simulink model "motor_model_9_az"  (R2018b)
settings: Solver=VariableStepAuto  StartTime=0.0  StopTime=1  RelTol=1e-7
model workspace (MAT data in the model file):
  A1 = 0.209333333333
  A2 = 0.0330526315789
  Ce = 0.27
  Cm = 0.36
  Jsumm = 7.5e-06
  K = 1000
  Kf = 0.1
  Km = 3.29
  Kn = 3.7
  L = 0.032
  Mn = 0.08
  R = 0.32
  T1 = 0.05
  T2 = 0.0001
  Te = 0.1
  Tm = 1.08
  Tpwm = 6.25e-05
  U = 27
  a = 0
  b = -2.09439510239
  c = 2.09439510239
  dt = 0.6
  dx = 3.14
  max = 3.14
  min = -3.14
  omega1 = 1.005
  omega2 = 6.28
  poles = 8
  target = 3.14
  w = 0.209333333333
libraries: simulink x2
settings Model: Creator=Sainquake  LastModifiedBy=Sainquake

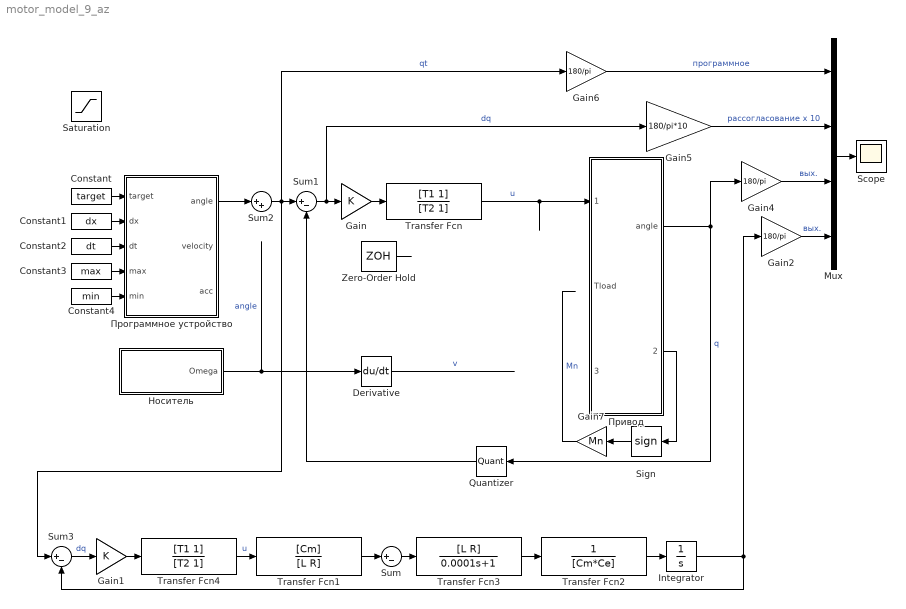
== system motor_model_9_az ==
  Constant : Constant  Value=target
  Constant1 : Constant  Value=dx
  Constant2 : Constant  Value=dt
  Constant3 : Constant  Value=max
  Constant4 : Constant  Value=min
  Derivative : Derivative
  Gain : Gain  Gain=K
  Gain1 : Gain  Gain=K
  Gain2 : Gain  Gain=180/pi
  Gain4 : Gain  Gain=180/pi
  Gain5 : Gain  Gain=180/pi*10
  Gain6 : Gain  Gain=180/pi
  Gain7 : Gain  Gain=Mn
  Integrator : Integrator
  Mux : Mux
  Quantizer : Quantizer  QuantizationInterval=0.0003
  Saturation : Saturate  UpperLimit=U/2  LowerLimit=-U/2
  Scope : Scope
  Sign : Signum  ZeroCross=off
  Sum : Sum  Inputs=|+-
  Sum1 : Sum  Inputs=|+-
  Sum2 : Sum  Inputs=|++
  Sum3 : Sum  Inputs=|+-
  Transfer Fcn : TransferFcn  Numerator=[T1 1]  Denominator=[T2 1]
  Transfer Fcn1 : TransferFcn  Numerator=[Cm]  Denominator=[L R]
  Transfer Fcn2 : TransferFcn  Numerator=1  Denominator=[Cm*Ce]
  Transfer Fcn3 : TransferFcn  Numerator=[L R]  Denominator=[0.0001 1]
  Transfer Fcn4 : TransferFcn  Numerator=[T1 1]  Denominator=[T2 1]
  Zero-Order Hold : ZeroOrderHold  SampleTime=Tpwm
  Носитель : Subsystem
  Привод : Subsystem
  Программное устройство : Subsystem
  wires:
  Sum1/1 -> Gain5/1, Gain/1  "dq"
  Sum2/1 -> Sum3/1, Gain6/1, Sum1/1  "qt"
  Привод/1(angle) -> Quantizer/1, Gain4/1  "q"
  Gain7/1 -> ?  "Mn"
  Носитель/1(Omega) -> Derivative/1  "angle"
  Constant/1 -> Программное устройство/1(target)
  Constant1/1 -> Программное устройство/2("dx ")
  Constant2/1 -> Программное устройство/3(dt)
  Constant4/1 -> Программное устройство/5(min)
  Constant3/1 -> Программное устройство/4(max)
  Gain/1 -> Transfer Fcn/1
  Gain4/1 -> Mux/3  "вых."
  Gain5/1 -> Mux/2  "рассогласование х 10"
  Gain6/1 -> Mux/1  "программное"
  Mux/1 -> Scope/1
  Transfer Fcn/1 -> Привод/1(target angle)  "u"
  Quantizer/1 -> Sum1/2
  Sign/1 -> Gain7/1
  Привод/2(velocity) -> Sign/1
  Программное устройство/1(angle) -> Sum2/1
  Zero-Order Hold/1 -> ?
  Derivative/1 -> ?  "v"
  Transfer Fcn1/1 -> Sum/1
  Transfer Fcn3/1 -> Transfer Fcn2/1
  Sum/1 -> Transfer Fcn3/1
  Transfer Fcn2/1 -> Integrator/1
  Gain1/1 -> Transfer Fcn4/1
  Transfer Fcn4/1 -> Transfer Fcn1/1  "u"
  Sum3/1 -> Gain1/1  "dq"
  Gain2/1 -> Mux/4  "вых."
  Integrator/1 -> Sum3/2, Gain2/1

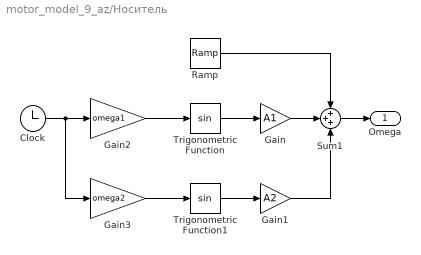
== system motor_model_9_az/Носитель ==
  Clock : Clock
  Gain : Gain  Gain=A1
  Gain1 : Gain  Gain=A2
  Gain2 : Gain  Gain=omega1
  Gain3 : Gain  Gain=omega2
  Ramp : simulink/Sources/Ramp  slope=w  start=0  InitialOutput=0
  Sum1 : Sum  Inputs=+++
  Trigonometric Function : Trigonometry
  Trigonometric Function1 : Trigonometry
  Omega : Outport
  wires:
  Trigonometric Function/1 -> Gain/1
  Trigonometric Function1/1 -> Gain1/1
  Clock/1 -> Gain2/1, Gain3/1
  Gain2/1 -> Trigonometric Function/1
  Gain3/1 -> Trigonometric Function1/1
  Gain/1 -> Sum1/2
  Gain1/1 -> Sum1/3
  Sum1/1 -> Omega/1
  Ramp/1 -> Sum1/1

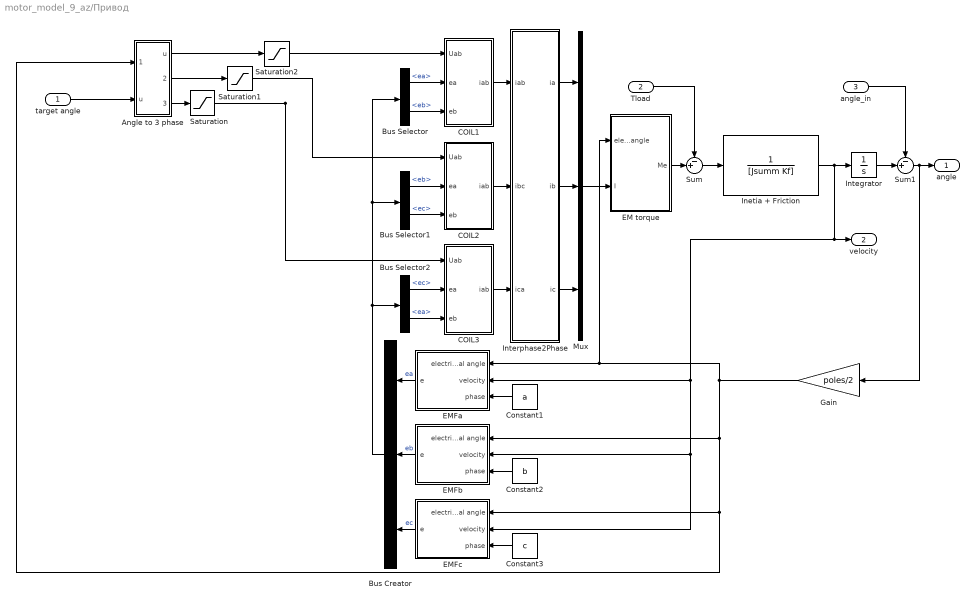
== system motor_model_9_az/Привод ==
  target angle : Inport
  Tload : Inport  Port=2
  angle_in : Inport  Port=3
  Angle to 3 phase : Subsystem
  Bus Creator : BusCreator  Inputs=3
  Bus Selector : BusSelector  OutputSignals=ea,eb
  Bus Selector1 : BusSelector  OutputSignals=eb,ec
  Bus Selector2 : BusSelector  OutputSignals=ec,ea
  COIL1 : Subsystem
  "COIL2 " : Subsystem
  COIL3 : Subsystem
  Constant1 : Constant  Value=a
  Constant2 : Constant  Value=b
  Constant3 : Constant  Value=c
  EM torque : Subsystem
  EMFa : Subsystem
  EMFb : Subsystem
  EMFc : Subsystem
  Gain : Gain  Gain=poles/2
  Inetia + Friction : TransferFcn  Denominator=[Jsumm Kf]
  Integrator : Integrator
  Interphase2Phase : Subsystem
  Mux : Mux  Inputs=3
  Saturation : Saturate  UpperLimit=U  LowerLimit=0
  Saturation1 : Saturate  UpperLimit=U  LowerLimit=0
  Saturation2 : Saturate  UpperLimit=U  LowerLimit=0
  Sum : Sum  Inputs=-+|
  Sum1 : Sum  Inputs=-+|
  angle : Outport
  velocity : Outport  Port=2
  wires:
  Tload/1 -> Sum/1
  Bus Creator/1 -> Bus Selector/1, Bus Selector1/1, Bus Selector2/1
  COIL1/1(iab) -> Interphase2Phase/1(iab)
  Interphase2Phase/1(ia) -> Mux/1
  Bus Selector2/2 -> COIL3/3(eb)  "<ea>"
  Gain/1 -> Angle to 3 phase/1(target), EMFc/1(electrical angle), EMFb/1(electrical angle), EM torque/1(electrical angle), EMFa/1(electrical angle)
  Bus Selector2/1 -> COIL3/2("ea ")  "<ec>"
  Bus Selector1/1 -> "COIL2 "/2("ea ")  "<eb>"
  Bus Selector1/2 -> "COIL2 "/3(eb)  "<ec>"
  Mux/1 -> EM torque/2(I)
  Bus Selector/2 -> COIL1/3(eb)  "<eb>"
  Bus Selector/1 -> COIL1/2("ea ")  "<ea>"
  Sum/1 -> Inetia + Friction/1
  Constant2/1 -> EMFb/3(phase)
  Constant3/1 -> EMFc/3(phase)
  Constant1/1 -> EMFa/3(phase)
  Inetia + Friction/1 -> Integrator/1, velocity/1, EMFc/2(velocity), EMFb/2(velocity), EMFa/2(velocity)
  EMFa/1(e) -> Bus Creator/1  "ea"
  EMFc/1(e) -> Bus Creator/3  "ec"
  EM torque/1(Me) -> Sum/2
  Interphase2Phase/3(ic) -> Mux/3
  "COIL2 "/1(iab) -> Interphase2Phase/2("ibc ")
  Angle to 3 phase/1("u ") -> Saturation2/1
  EMFb/1(e) -> Bus Creator/2  "eb"
  Angle to 3 phase/3(u 2) -> Saturation/1
  Angle to 3 phase/2(u 1) -> Saturation1/1
  Interphase2Phase/2(ib) -> Mux/2
  COIL3/1(iab) -> Interphase2Phase/3(ica)
  angle_in/1 -> Sum1/1
  Integrator/1 -> Sum1/2
  target angle/1 -> Angle to 3 phase/2(u)
  Sum1/1 -> angle/1, Gain/1
  Saturation2/1 -> COIL1/1(Uab)
  Saturation1/1 -> "COIL2 "/1(Uab)
  Saturation/1 -> COIL3/1(Uab)

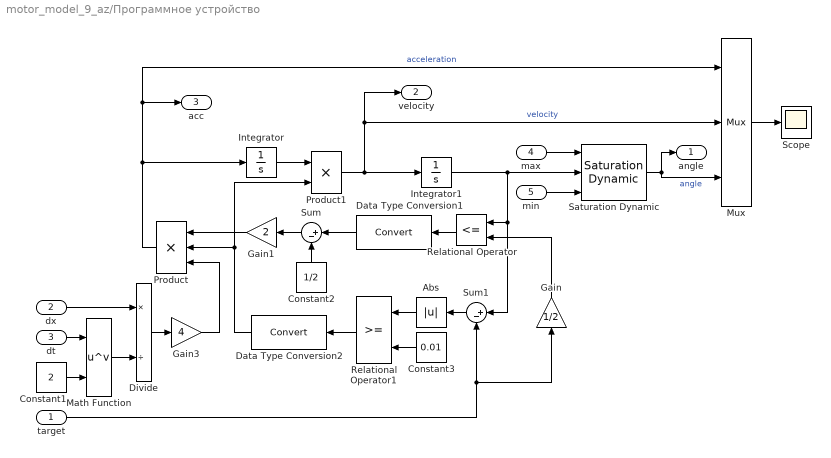
== system motor_model_9_az/Программное устройство ==
  target : Inport
  "dx " : Inport  Port=2
  dt : Inport  Port=3
  max : Inport  Port=4
  min : Inport  Port=5
  Abs : Abs
  Constant1 : Constant  Value=2
  Constant2 : Constant  Value=1/2
  Constant3 : Constant  Value=0.01
  Data Type Conversion1 : DataTypeConversion
  Data Type Conversion2 : DataTypeConversion
  Divide : Product  Inputs=*/
  Gain : Gain  Gain=1/2
  Gain1 : Gain  Gain=2
  Gain3 : Gain  Gain=4
  Integrator : Integrator
  Integrator1 : Integrator
  Math Function : Math  Operator=pow  SaturateOnIntegerOverflow=on
  Mux : Mux  Inputs=3
  Product : Product  Inputs=3
  Product1 : Product
  Relational Operator : RelationalOperator  Operator=<=  OutDataTypeStr=boolean  RndMeth=Simplest
  Relational Operator1 : RelationalOperator  OutDataTypeStr=boolean  RndMeth=Simplest
  Saturation Dynamic : simulink/Discontinuities/Saturation Dynamic  OutMin=[]  OutMax=[]  OutDataTypeStr=Inherit: Same as second input  OutDataType=fixdt(1, 16)  OutScaling=2^-10  DoSatur=off
  Scope : Scope
  Sum : Sum  Inputs=|+-
  Sum1 : Sum  Inputs=|+-
  angle : Outport
  velocity : Outport  Port=2
  acc : Outport  Port=3
  wires:
  "dx "/1 -> Divide/1
  Constant1/1 -> Math Function/2
  Gain3/1 -> Product/3
  Data Type Conversion1/1 -> Sum/1
  Sum/1 -> Gain1/1
  Product/1 -> Integrator/1, Mux/1, acc/1  "acceleration"
  Product1/1 -> Integrator1/1, Mux/2, velocity/1  "velocity"
  Abs/1 -> Relational Operator1/1
  Relational Operator1/1 -> Data Type Conversion2/1
  Sum1/1 -> Abs/1
  Data Type Conversion2/1 -> Product1/2, Product/2
  Divide/1 -> Gain3/1
  Constant2/1 -> Sum/2
  Integrator/1 -> Product1/1
  target/1 -> Gain/1, Sum1/2
  Math Function/1 -> Divide/2
  Gain/1 -> Relational Operator/2
  Integrator1/1 -> Sum1/1, Relational Operator/1, Saturation Dynamic/2
  Mux/1 -> Scope/1
  Gain1/1 -> Product/1
  Relational Operator/1 -> Data Type Conversion1/1
  dt/1 -> Math Function/1
  Constant3/1 -> Relational Operator1/2
  max/1 -> Saturation Dynamic/1
  min/1 -> Saturation Dynamic/3
  Saturation Dynamic/1 -> Mux/3, angle/1  "angle"

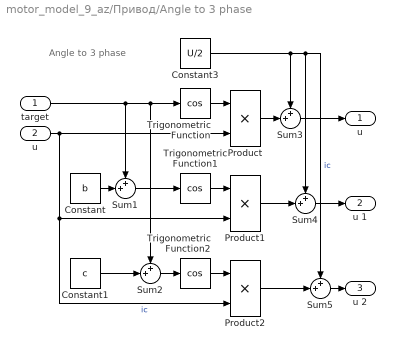
== system motor_model_9_az/Привод/Angle to 3 phase ==
  note: Angle to 3 phase
  target : Inport
  u : Inport  Port=2
  Constant : Constant  Value=b
  Constant1 : Constant  Value=c
  Constant3 : Constant  Value=U/2
  Product : Product
  Product1 : Product
  Product2 : Product
  Sum{1..5} (5 alike) : Sum  Inputs=++|
  Trigonometric Function : Trigonometry  Operator=cos
  Trigonometric Function1 : Trigonometry  Operator=cos
  Trigonometric Function2 : Trigonometry  Operator=cos
  "u " : Outport
  u 1 : Outport  Port=2
  u 2 : Outport  Port=3
  wires:
  Sum3/1 -> "u "/1
  target/1 -> Sum2/1, Trigonometric Function/1, Sum1/1
  Trigonometric Function2/1 -> Product2/1
  Sum2/1 -> Trigonometric Function2/1
  Trigonometric Function1/1 -> Product1/1
  u/1 -> Product/2, Product2/2, Product1/2  "ic"
  Constant1/1 -> Sum2/2
  Sum1/1 -> Trigonometric Function1/1
  Constant/1 -> Sum1/2
  Trigonometric Function/1 -> Product/1
  Constant3/1 -> Sum5/1, Sum4/1, Sum3/1  "ic"
  Product/1 -> Sum3/2
  Product1/1 -> Sum4/2
  Product2/1 -> Sum5/2
  Sum5/1 -> u 2/1
  Sum4/1 -> u 1/1

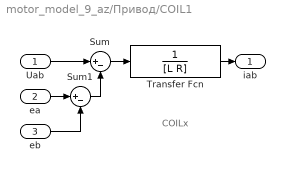
== system motor_model_9_az/Привод/COIL1 ==
  note: COILx
  Uab : Inport
  "ea " : Inport  Port=2
  eb : Inport  Port=3
  Sum : Sum  Inputs=|+-
  Sum1 : Sum  Inputs=|+-
  Transfer Fcn : TransferFcn  Denominator=[L R]
  iab : Outport
  wires:
  Uab/1 -> Sum/1
  Transfer Fcn/1 -> iab/1
  Sum/1 -> Transfer Fcn/1
  "ea "/1 -> Sum1/1
  eb/1 -> Sum1/2
  Sum1/1 -> Sum/2

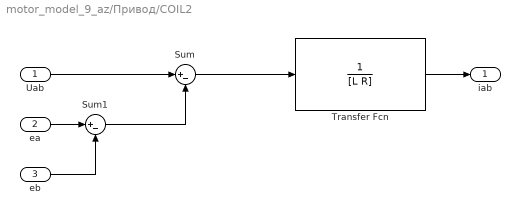
== system motor_model_9_az/Привод/COIL2  ==
  Uab : Inport
  "ea " : Inport  Port=2
  eb : Inport  Port=3
  Sum : Sum  Inputs=|+-
  Sum1 : Sum  Inputs=|+-
  Transfer Fcn : TransferFcn  Denominator=[L R]
  iab : Outport
  wires:
  Uab/1 -> Sum/1
  Transfer Fcn/1 -> iab/1
  Sum/1 -> Transfer Fcn/1
  "ea "/1 -> Sum1/1
  eb/1 -> Sum1/2
  Sum1/1 -> Sum/2

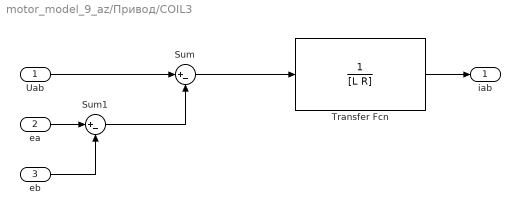
== system motor_model_9_az/Привод/COIL3 ==
  Uab : Inport
  "ea " : Inport  Port=2
  eb : Inport  Port=3
  Sum : Sum  Inputs=|+-
  Sum1 : Sum  Inputs=|+-
  Transfer Fcn : TransferFcn  Denominator=[L R]
  iab : Outport
  wires:
  Uab/1 -> Sum/1
  Transfer Fcn/1 -> iab/1
  Sum/1 -> Transfer Fcn/1
  "ea "/1 -> Sum1/1
  eb/1 -> Sum1/2
  Sum1/1 -> Sum/2

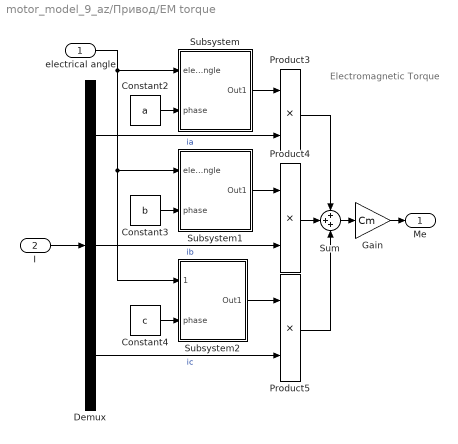
== system motor_model_9_az/Привод/EM torque ==
  note: Electromagnetic Torque
  electrical angle : Inport
  I : Inport  Port=2
  Constant2 : Constant  Value=a
  Constant3 : Constant  Value=b
  Constant4 : Constant  Value=c
  Demux : Demux  Outputs=3
  Gain : Gain  Gain=Cm
  Product3 : Product
  Product4 : Product
  Product5 : Product
  Subsystem : Subsystem
  Subsystem1 : Subsystem
  Subsystem2 : Subsystem
  Sum : Sum  Inputs=+++
  Me : Outport
  wires:
  Sum/1 -> Gain/1
  Gain/1 -> Me/1
  I/1 -> Demux/1
  Constant2/1 -> Subsystem/2(phase)
  electrical angle/1 -> Subsystem2/1(electrical angle), Subsystem1/1(electrical angle), Subsystem/1(electrical angle)
  Constant3/1 -> Subsystem1/2(phase)
  Constant4/1 -> Subsystem2/2(phase)
  Demux/1 -> Product3/2  "ia"
  Subsystem/1(Out1) -> Product3/1
  Demux/2 -> Product4/2  "ib"
  Demux/3 -> Product5/2  "ic"
  Subsystem1/1(Out1) -> Product4/1
  Subsystem2/1(Out1) -> Product5/1
  Product4/1 -> Sum/2
  Product3/1 -> Sum/1
  Product5/1 -> Sum/3

== system motor_model_9_az/Привод/EMFa ==
  note: EMF
  electrical angle : Inport
  velocity : Inport  Port=2
  phase : Inport  Port=3
  Gain : Gain  Gain=Ce
  Product1 : Product
  Subsystem : Subsystem
  e : Outport
  wires:
  Gain/1 -> Product1/2
  Product1/1 -> e/1
  velocity/1 -> Gain/1
  phase/1 -> Subsystem/2(phase)
  electrical angle/1 -> Subsystem/1(electrical angle)
  Subsystem/1(Out1) -> Product1/1

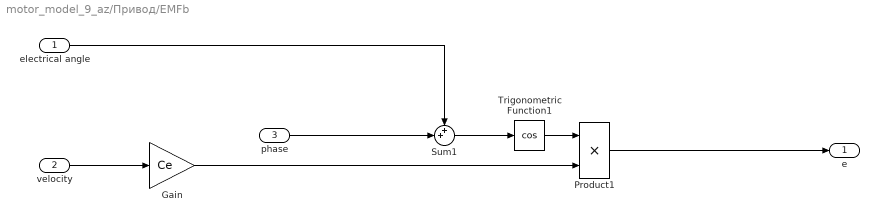
== system motor_model_9_az/Привод/EMFb ==
  electrical angle : Inport
  velocity : Inport  Port=2
  phase : Inport  Port=3
  Gain : Gain  Gain=Ce
  Product1 : Product
  Sum1 : Sum  Inputs=++|
  Trigonometric Function1 : Trigonometry  Operator=cos
  e : Outport
  wires:
  Trigonometric Function1/1 -> Product1/1
  Gain/1 -> Product1/2
  Sum1/1 -> Trigonometric Function1/1
  phase/1 -> Sum1/2
  electrical angle/1 -> Sum1/1
  Product1/1 -> e/1
  velocity/1 -> Gain/1

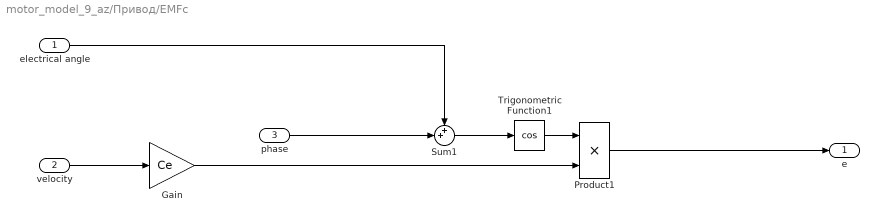
== system motor_model_9_az/Привод/EMFc ==
  electrical angle : Inport
  velocity : Inport  Port=2
  phase : Inport  Port=3
  Gain : Gain  Gain=Ce
  Product1 : Product
  Sum1 : Sum  Inputs=++|
  Trigonometric Function1 : Trigonometry  Operator=cos
  e : Outport
  wires:
  Trigonometric Function1/1 -> Product1/1
  Gain/1 -> Product1/2
  Sum1/1 -> Trigonometric Function1/1
  phase/1 -> Sum1/2
  electrical angle/1 -> Sum1/1
  Product1/1 -> e/1
  velocity/1 -> Gain/1

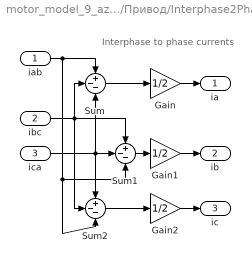
== system motor_model_9_az/Привод/Interphase2Phase ==
  note: Interphase to phase currents
  iab : Inport
  "ibc " : Inport  Port=2
  ica : Inport  Port=3
  Gain : Gain  Gain=1/2
  Gain1 : Gain  Gain=1/2
  Gain2 : Gain  Gain=1/2
  Sum : Sum  Inputs=+--
  Sum1 : Sum  Inputs=+--
  Sum2 : Sum  Inputs=+--
  ia : Outport
  ib : Outport  Port=2
  ic : Outport  Port=3
  wires:
  Gain/1 -> ia/1
  Gain1/1 -> ib/1
  Gain2/1 -> ic/1
  iab/1 -> Sum2/3, Sum1/3, Sum/1
  "ibc "/1 -> Sum2/2, Sum1/1, Sum/2
  ica/1 -> Sum/3, Sum2/1, Sum1/2
  Sum/1 -> Gain/1
  Sum1/1 -> Gain1/1
  Sum2/1 -> Gain2/1

== system motor_model_9_az/Привод/EM torque/Subsystem ==
  electrical angle : Inport
  phase : Inport  Port=2
  Sum1 : Sum  Inputs=++|
  Trigonometric Function1 : Trigonometry  Operator=cos
  Out1 : Outport
  wires:
  electrical angle/1 -> Sum1/1
  Sum1/1 -> Trigonometric Function1/1
  phase/1 -> Sum1/2
  Trigonometric Function1/1 -> Out1/1

== system motor_model_9_az/Привод/EM torque/Subsystem1 ==
  electrical angle : Inport
  phase : Inport  Port=2
  Sum1 : Sum  Inputs=++|
  Trigonometric Function1 : Trigonometry  Operator=cos
  Out1 : Outport
  wires:
  electrical angle/1 -> Sum1/1
  Sum1/1 -> Trigonometric Function1/1
  phase/1 -> Sum1/2
  Trigonometric Function1/1 -> Out1/1

== system motor_model_9_az/Привод/EM torque/Subsystem2 ==
  electrical angle : Inport
  phase : Inport  Port=2
  Sum1 : Sum  Inputs=++|
  Trigonometric Function1 : Trigonometry  Operator=cos
  Out1 : Outport
  wires:
  electrical angle/1 -> Sum1/1
  Sum1/1 -> Trigonometric Function1/1
  phase/1 -> Sum1/2
  Trigonometric Function1/1 -> Out1/1

== system motor_model_9_az/Привод/EMFa/Subsystem ==
  electrical angle : Inport
  phase : Inport  Port=2
  Sum1 : Sum  Inputs=++|
  Trigonometric Function1 : Trigonometry  Operator=cos
  Out1 : Outport
  wires:
  electrical angle/1 -> Sum1/1
  Sum1/1 -> Trigonometric Function1/1
  phase/1 -> Sum1/2
  Trigonometric Function1/1 -> Out1/1
